simulink model "pitch_lineal"  (R2015a)
settings: Solver=ode45  StartTime=0.0  StopTime=28.0  RelTol=1e-3
values from neighbouring files (symbols this model uses):
  Kpitch = 2*l*Ktheta*Kt/Iyy    (= 114.333391207)    [Parametros.m]
  tau = 0.06035    [Parametros.m]
libraries: simulink x5
settings Model: Creator=simaqtel  LastModifiedBy=Eduardo

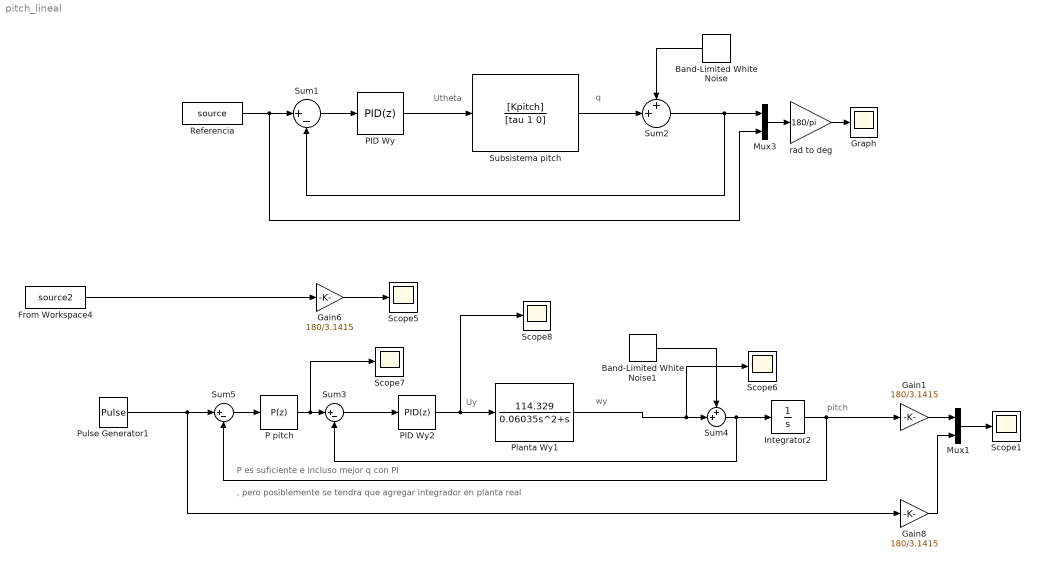
== system pitch_lineal ==
  note: , pero posiblemente se tendra que agregar integrador en planta real
  note: P es suficiente e incluso mejor q con PI
  note: pitch
  note: q
  note: Utheta
  note: wy
  note: Uy
  Band-Limited White Noise : simulink/Sources/Band-Limited White Noise  Cov=[0.000001]  Ts=0.01  seed=[23341]
  Band-Limited White Noise1 : simulink/Sources/Band-Limited White Noise  Cov=[0.000001]  Ts=0.01  seed=[23341]
  From Workspace4 : FromWorkspace  VariableName=source2  SampleTime=0.01
  Gain1 : Gain  Gain=180/3.1415
  Gain6 : Gain  Gain=180/3.1415
  Gain8 : Gain  Gain=180/3.1415
  Graph : Scope
      settings: SaveName=ScopeData3
  Integrator2 : Integrator
  Mux1 : Mux  Inputs=2
  Mux3 : Mux  Inputs=2
  P pitch : simulink/Continuous/PID Controller  Controller=P  TimeDomain=Discrete-time  SampleTime=0.01  IntegratorMethod=Forward Euler  FilterMethod=Forward Euler  Form=Parallel  UseFilter=off  ControllerParametersSource=internal  P=6.15  I=0.5  D=0.05  N=20.2444442041031  InitialConditionSource=internal  InitialConditionForIntegrator=0  InitialConditionForFilter=0  ExternalReset=none  LimitOutput=off  UpperSaturationLimit=3  LowerSaturationLimit=-3  LinearizeAsGain=on  AntiWindupMode=none  Kb=1  TrackingMode=off  Kt=1  PParamMin=[]  PParamMax=[]  IParamMin=[]  IParamMax=[]  DParamMin=[]  DParamMax=[]  NParamMin=[]  NParamMax=[]  KbParamMin=[]  KbParamMax=[]  KtParamMin=[]  KtParamMax=[]  POutMin=[]  POutMax=[]  IOutMin=[]  IOutMax=[]  DOutMin=[]  DOutMax=[]  NOutMin=[]  NOutMax=[]  KbOutMin=[]  KbOutMax=[]  KtOutMin=[]  KtOutMax=[]  IntegratorOutMin=[]  IntegratorOutMax=[]  FilterOutMin=[]  FilterOutMax=[]  SumOutMin=[]  SumOutMax=[]  SumI1OutMin=[]  SumI1OutMax=[]  SumI2OutMin=[]  SumI2OutMax=[]  SumI3OutMin=[]  SumI3OutMax=[]  SumDOutMin=[]  SumDOutMax=[]  SaturationOutMin=[]  SaturationOutMax=[]  IntegratorContinuousStateAttributes=''  IntegratorStateMustResolveToSignalObject=off  IntegratorRTWStateStorageClass=Auto  FilterContinuousStateAttributes=''  FilterStateMustResolveToSignalObject=off  FilterRTWStateStorageClass=Auto  DifferentiatorICPrevScaledInput=0  DifferentiatorOutMin=[]  DifferentiatorOutMax=[]
  PID Wy : simulink/Continuous/PID Controller  Controller=PID  TimeDomain=Discrete-time  SampleTime=0.01  IntegratorMethod=Forward Euler  FilterMethod=Forward Euler  Form=Ideal  UseFilter=on  ControllerParametersSource=internal  P=0.186108527660047  I=0.270831955527183  D=0.0957187049121133  N=189.58120119176  InitialConditionSource=internal  InitialConditionForIntegrator=0  InitialConditionForFilter=0  ExternalReset=none  LimitOutput=on  UpperSaturationLimit=1  LowerSaturationLimit=-1  LinearizeAsGain=on  AntiWindupMode=back-calculation  Kb=1  TrackingMode=off  Kt=1  PParamMin=[]  PParamMax=[]  IParamMin=[]  IParamMax=[]  DParamMin=[]  DParamMax=[]  NParamMin=[]  NParamMax=[]  KbParamMin=[]  KbParamMax=[]  KtParamMin=[]  KtParamMax=[]  POutMin=[]  POutMax=[]  IOutMin=[]  IOutMax=[]  DOutMin=[]  DOutMax=[]  NOutMin=[]  NOutMax=[]  KbOutMin=[]  KbOutMax=[]  KtOutMin=[]  KtOutMax=[]  IntegratorOutMin=[]  IntegratorOutMax=[]  FilterOutMin=[]  FilterOutMax=[]  SumOutMin=[]  SumOutMax=[]  SumI1OutMin=[]  SumI1OutMax=[]  SumI2OutMin=[]  SumI2OutMax=[]  SumI3OutMin=[]  SumI3OutMax=[]  SumDOutMin=[]  SumDOutMax=[]  SaturationOutMin=[]  SaturationOutMax=[]  IntegratorContinuousStateAttributes=''  IntegratorStateMustResolveToSignalObject=off  IntegratorRTWStateStorageClass=Auto  FilterContinuousStateAttributes=''  FilterStateMustResolveToSignalObject=off  FilterRTWStateStorageClass=Auto  DifferentiatorICPrevScaledInput=0  DifferentiatorOutMin=[]  DifferentiatorOutMax=[]
  PID Wy2 : simulink/Continuous/PID Controller  Controller=PID  TimeDomain=Discrete-time  SampleTime=0.01  IntegratorMethod=Forward Euler  FilterMethod=Forward Euler  Form=Ideal  UseFilter=on  ControllerParametersSource=internal  P=0.186108527660047  I=0.270831955527183  D=0.0957187049121133  N=189.58120119176  InitialConditionSource=internal  InitialConditionForIntegrator=0  InitialConditionForFilter=0  ExternalReset=none  LimitOutput=on  UpperSaturationLimit=1  LowerSaturationLimit=-1  LinearizeAsGain=on  AntiWindupMode=back-calculation  Kb=1  TrackingMode=off  Kt=1  PParamMin=[]  PParamMax=[]  IParamMin=[]  IParamMax=[]  DParamMin=[]  DParamMax=[]  NParamMin=[]  NParamMax=[]  KbParamMin=[]  KbParamMax=[]  KtParamMin=[]  KtParamMax=[]  POutMin=[]  POutMax=[]  IOutMin=[]  IOutMax=[]  DOutMin=[]  DOutMax=[]  NOutMin=[]  NOutMax=[]  KbOutMin=[]  KbOutMax=[]  KtOutMin=[]  KtOutMax=[]  IntegratorOutMin=[]  IntegratorOutMax=[]  FilterOutMin=[]  FilterOutMax=[]  SumOutMin=[]  SumOutMax=[]  SumI1OutMin=[]  SumI1OutMax=[]  SumI2OutMin=[]  SumI2OutMax=[]  SumI3OutMin=[]  SumI3OutMax=[]  SumDOutMin=[]  SumDOutMax=[]  SaturationOutMin=[]  SaturationOutMax=[]  IntegratorContinuousStateAttributes=''  IntegratorStateMustResolveToSignalObject=off  IntegratorRTWStateStorageClass=Auto  FilterContinuousStateAttributes=''  FilterStateMustResolveToSignalObject=off  FilterRTWStateStorageClass=Auto  DifferentiatorICPrevScaledInput=0  DifferentiatorOutMin=[]  DifferentiatorOutMax=[]
  Planta Wy1 : TransferFcn  Numerator=[114.329]  Denominator=[0.06035 1 0]
  Pulse Generator1 : DiscretePulseGenerator  PulseType=Time based  Amplitude=0.3  Period=9  PulseWidth=55  PhaseDelay=4
  Referencia : FromWorkspace  VariableName=source  SampleTime=0.01
  Scope{1,5..8} (5 alike) : Scope
      Scope1 settings: TimeRange=1.085807108091082  YMin=-1.321354166666669  YMax=18.16197916666667
      Scope5 settings: SaveName=ScopeData5
      Scope7 settings: SaveName=ScopeData6
      Scope8 settings: SaveName=ScopeData7
  Subsistema pitch : TransferFcn  Numerator=[Kpitch]  Denominator=[tau 1 0]
  Sum1 : Sum  Inputs=|+-
  Sum2 : Sum  Inputs=++|
  Sum3 : Sum  Inputs=|+-
  Sum4 : Sum  Inputs=++|
  Sum5 : Sum  Inputs=|+-
  rad to deg : Gain  Gain=180/pi
  wires:
  Sum1/1 -> PID Wy/1
  From Workspace4/1 -> Gain6/1
  Sum2/1 -> Sum1/2, Mux3/1
  Subsistema pitch/1 -> Sum2/2
  Band-Limited White Noise/1 -> Sum2/1
  Gain6/1 -> Scope5/1
  Mux1/1 -> Scope1/1
  Gain1/1 -> Mux1/1
  Sum4/1 -> Integrator2/1, Sum3/2
  Planta Wy1/1 -> Scope6/1, Sum4/2
  Band-Limited White Noise1/1 -> Sum4/1
  Gain8/1 -> Mux1/2
  P pitch/1 -> Scope7/1, Sum3/1
  Sum5/1 -> P pitch/1
  Pulse Generator1/1 -> Gain8/1, Sum5/1
  Integrator2/1 -> Gain1/1, Sum5/2
  Referencia/1 -> Mux3/2, Sum1/1
  PID Wy/1 -> Subsistema pitch/1
  PID Wy2/1 -> Scope8/1, Planta Wy1/1
  Sum3/1 -> PID Wy2/1
  Mux3/1 -> rad to deg/1
  rad to deg/1 -> Graph/1
